simulink model "HVAC"  (R2021a)
settings: Solver=FixedStepAuto  StartTime=0.0  StopTime=1400  FixedStep=1  RelTol=1e-3
values from neighbouring files (symbols this model uses):
  A_w = 1.73    [HVAC_Modeling.m]
  ACCOP = 2.4    [HVAC_Modeling.m]
  AMH = 55    [HVAC_Modeling.m]
  Av = 7.87    [HVAC_Modeling.m]
  c = 1350    [HVAC_Modeling.m]
  Distance = 5.303    [HVAC_Modeling.m]
  h_c = data(2,2:7)    [HVAC_Modeling.m]
  h_v = data(1,2:7)    [HVAC_Modeling.m]
  HCOP = 1    [HVAC_Modeling.m]
  Height = 1.6    [HVAC_Modeling.m]
  m = 0.035    [HVAC_Modeling.m]
  m_a = 0.4    [HVAC_Modeling.m]
  M_a = 3.185    [HVAC_Modeling.m]
  n = 1    [HVAC_Modeling.m]
  R_solar = 0    [HVAC_Modeling.m]
  Tamb = NLT_tem_c(i)    [HVAC_Modeling.m]
  Tc = 23    [HVAC_Modeling.m]
  Ti = NLT_tem_c(i)    [HVAC_Modeling.m]
  Trans = 0.4    [HVAC_Modeling.m]
  Weight = 70    [HVAC_Modeling.m]
settings Model: Creator=LENOVO  LastModifiedBy=LENOVO

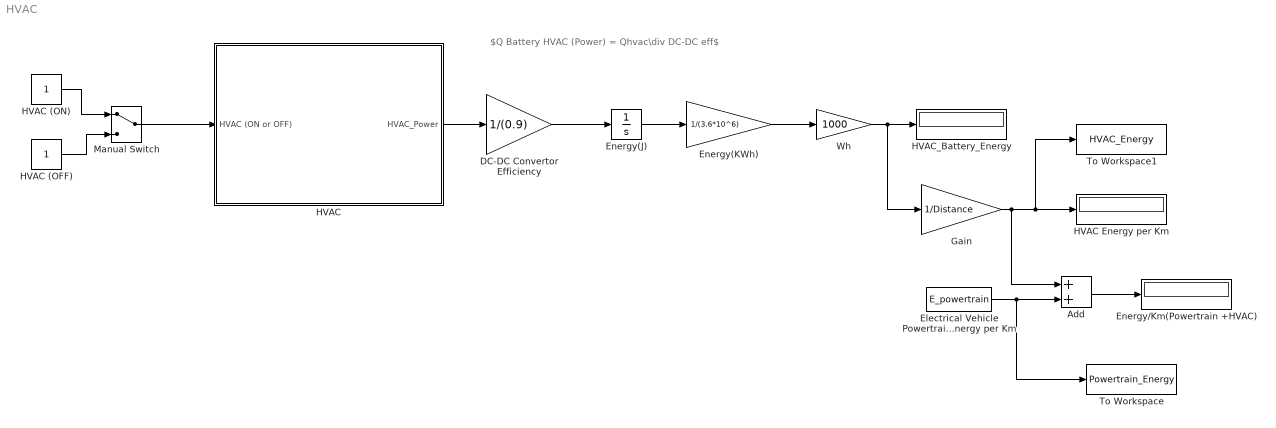
== system HVAC ==
  note: $Q Battery HVAC (Power) = Qhvac\div DC-DC eff$
  Add : Sum
  DC-DC Convertor Efficiency : Gain  Gain=1/(0.9)
  "Electrical Vehicle Powertrain Energy per Km " : FromWorkspace  VariableName=E_powertrain
  Energy(J) : Integrator
  Energy(KWh) : Gain  Gain=1/(3.6*10^6)
  Energy/Km(Powertrain +HVAC) : Display
  Gain : Gain  Gain=1/Distance
  HVAC : Subsystem
  HVAC (OFF) : Constant
  HVAC (ON) : Constant
  HVAC Energy per Km : Display
  HVAC_Battery_Energy : Display
  Manual Switch : ManualSwitch
  To Workspace : ToWorkspace  VariableName=Powertrain_Energy  SaveFormat=Timeseries  SampleTime=-1
  To Workspace1 : ToWorkspace  VariableName=HVAC_Energy  SaveFormat=Timeseries  SampleTime=-1
  Wh : Gain  Gain=1000
  wires:
  HVAC/1(HVAC_Power) -> DC-DC Convertor Efficiency/1
  DC-DC Convertor Efficiency/1 -> Energy(J)/1
  Energy(J)/1 -> Energy(KWh)/1
  Energy(KWh)/1 -> Wh/1
  Wh/1 -> Gain/1, HVAC_Battery_Energy/1
  Gain/1 -> Add/1, To Workspace1/1, HVAC Energy per Km/1
  "Electrical Vehicle Powertrain Energy per Km "/1 -> To Workspace/1, Add/2
  Add/1 -> Energy/Km(Powertrain +HVAC)/1
  Manual Switch/1 -> HVAC/1(HVAC (ON or OFF))
  HVAC (ON)/1 -> Manual Switch/1
  HVAC (OFF)/1 -> Manual Switch/2

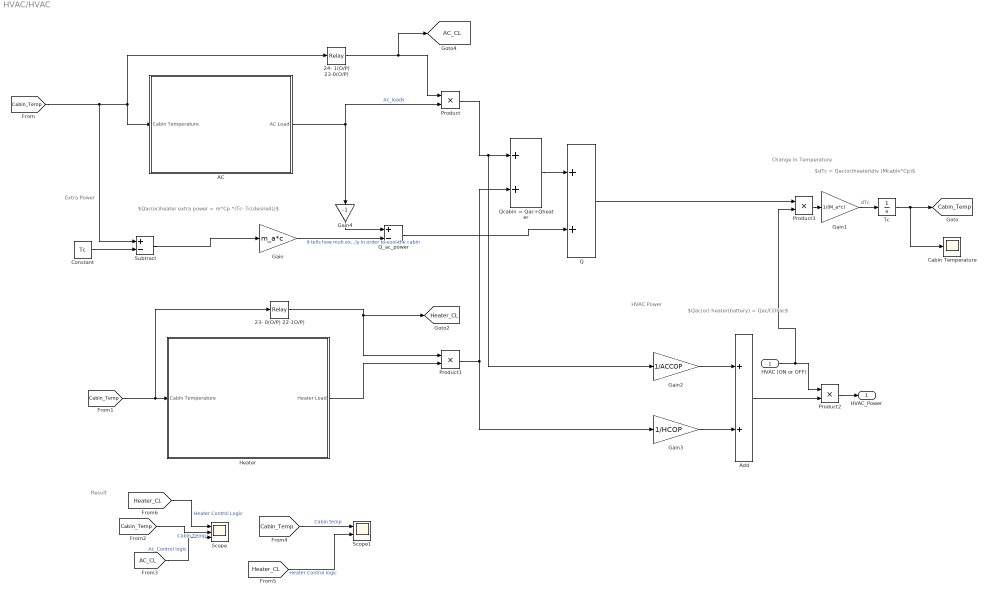
== system HVAC/HVAC ==
  note: HVAC Power
  note: $Qac(or) heater(battery) = Qac/COPac$
  note: Result
  note: Change in Temperature
  note: Extra Power
  note: $dTc = Qac(or)heater\div (Mcabin*Cp)$
  note: $Qac(or)heater extra power = m*Cp *(Tc- Tc(desired))$
  HVAC (ON or OFF) : Inport
  23- 0(O/P) 22-1O/P) : Relay  OnSwitchValue=Tc  OffSwitchValue=Tc-1  OnOutputValue=0  OffOutputValue=1
  24- 1(O/P) 23-0(O/P) : Relay  OnSwitchValue=Tc+1  OffSwitchValue=Tc
  AC : Subsystem
  Add : Sum
  Cabin Temperature : Scope
  Constant : Constant  Value=Tc
  Gain : Gain  Gain=m_a*c
  Gain1 : Gain  Gain=1/(M_a*c)
  Gain2 : Gain  Gain=1/ACCOP
  Gain3 : Gain  Gain=1/HCOP
  Gain4 : Gain  Gain=-1
  Heater : Subsystem
  Product{,1..3} (4 alike) : Product
  Q : Sum
  Q_ac_power : Sum  Inputs=+-
  Qcabin = Qac+Qheater : Sum
  Scope : Scope  NumInputPorts=3
  Scope1 : Scope  NumInputPorts=2
  Subtract : Sum  Inputs=+-
  Tc : Integrator  InitialCondition=Ti
  HVAC_Power : Outport
  tag scope: AC_CL=global, Cabin_Temp=global, Heater_CL=global
  wires:
  Constant/1 -> Subtract/2
  Subtract/1 -> Gain/1
  Gain/1 -> Q_ac_power/2  "It tells how muh extra power need to supply in order to cool the cabin"
  AC/1(AC Load) -> Product/2, Gain4/1  "Ac_loads"
  Gain1/1 -> Tc/1  "dTc"
  [Cabin_Temp] -> AC/1(Cabin Temperature), 24- 1(O/P) 23-0(O/P)/1, Subtract/1
  [Cabin_Temp] -> 23- 0(O/P) 22-1O/P)/1, Heater/1(Cabin Temperature)
  24- 1(O/P) 23-0(O/P)/1 -> [AC_CL], Product/1
  23- 0(O/P) 22-1O/P)/1 -> Product1/1, [Heater_CL]
  Heater/1(Heater Load) -> Product1/2
  Product/1 -> Qcabin = Qac+Qheater/1, Gain2/1
  Qcabin = Qac+Qheater/1 -> Q/1
  Q_ac_power/1 -> Q/2
  Tc/1 -> Cabin Temperature/1, [Cabin_Temp]
  [Cabin_Temp] -> Scope/2  "Cabin Temp"
  [AC_CL] -> Scope/3  "Ac_Control logic"
  [Cabin_Temp] -> Scope1/1  "Cabin temp"
  [Heater_CL] -> Scope1/2  "Heater Control logic"
  Product1/1 -> Gain3/1, Qcabin = Qac+Qheater/2
  Gain2/1 -> Add/1
  Gain3/1 -> Add/2
  Gain4/1 -> Q_ac_power/1
  Add/1 -> Product2/2
  HVAC (ON or OFF)/1 -> Product3/2, Product2/1
  Product2/1 -> HVAC_Power/1
  Product3/1 -> Gain1/1
  Q/1 -> Product3/1
  [Heater_CL] -> Scope/1  "Heater Control Logic"

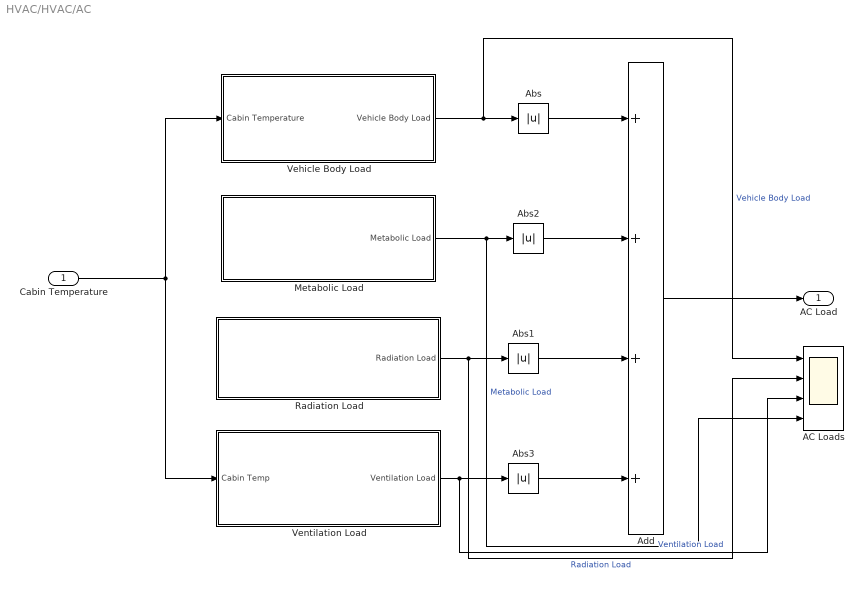
== system HVAC/HVAC/AC ==
  Cabin Temperature : Inport
  AC Loads : Scope  NumInputPorts=4
  Abs{,1..3} (4 alike) : Abs
  Add : Sum  Inputs=++++
  Metabolic Load : Subsystem
  Radiation Load : Subsystem
  Vehicle Body Load : Subsystem
  Ventilation Load : Subsystem
  AC Load : Outport
  wires:
  Cabin Temperature/1 -> Vehicle Body Load/1(Cabin Temperature), Ventilation Load/1(Cabin Temp)
  Metabolic Load/1(Metabolic Load) -> AC Loads/4, Abs2/1  "Metabolic Load"
  Add/1 -> AC Load/1
  Vehicle Body Load/1(Vehicle Body Load) -> AC Loads/1, Abs/1  "Vehicle Body Load"
  Abs/1 -> Add/1
  Abs2/1 -> Add/2
  Radiation Load/1(Radiation Load) -> AC Loads/2, Abs1/1  "Radiation Load"
  Abs1/1 -> Add/3
  Ventilation Load/1(Ventilation Load) -> AC Loads/3, Abs3/1  "Ventilation Load"
  Abs3/1 -> Add/4

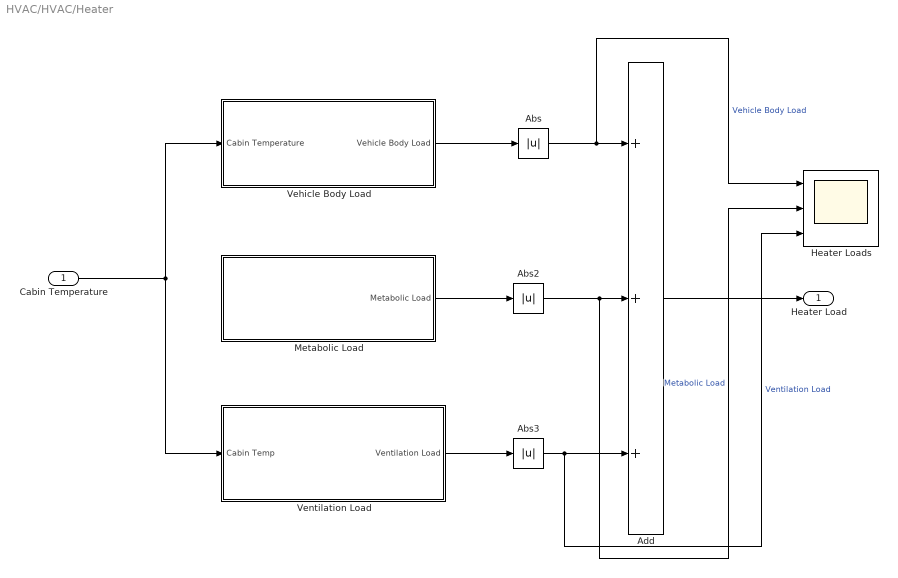
== system HVAC/HVAC/Heater ==
  Cabin Temperature : Inport
  Abs : Abs
  Abs2 : Abs
  Abs3 : Abs
  Add : Sum  Inputs=+++
  Heater Loads : Scope  NumInputPorts=3
  Metabolic Load : Subsystem
  Vehicle Body Load : Subsystem
  Ventilation Load : Subsystem
  Heater Load : Outport
  wires:
  Cabin Temperature/1 -> Vehicle Body Load/1(Cabin Temperature), Ventilation Load/1(Cabin Temp)
  Metabolic Load/1(Metabolic Load) -> Abs2/1
  Add/1 -> Heater Load/1
  Vehicle Body Load/1(Vehicle Body Load) -> Abs/1
  Abs/1 -> Heater Loads/1, Add/1  "Vehicle Body Load"
  Abs2/1 -> Heater Loads/2, Add/2  "Metabolic Load"
  Ventilation Load/1(Ventilation Load) -> Abs3/1
  Abs3/1 -> Heater Loads/3, Add/3  "Ventilation Load"

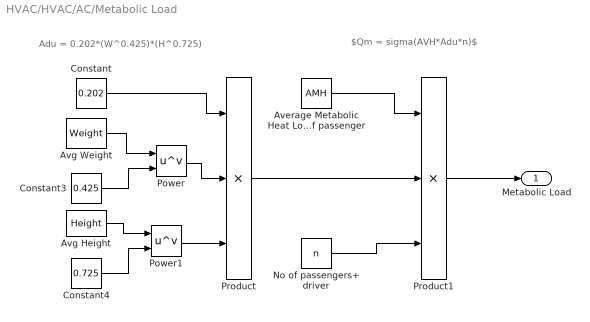
== system HVAC/HVAC/AC/Metabolic Load ==
  note: Adu = 0.202*(W^0.425)*(H^0.725)
  note: $Qm = sigma(AVH*Adu*n)$
  Average Metabolic Heat Load of passenger : Constant  Value=AMH
  Avg Height : Constant  Value=Height
  Avg Weight : Constant  Value=Weight
  Constant : Constant  Value=0.202
  Constant3 : Constant  Value=0.425
  Constant4 : Constant  Value=0.725
  "No of passengers+ driver " : Constant  Value=n
  Power : Math  Operator=pow  SaturateOnIntegerOverflow=on
  Power1 : Math  Operator=pow  SaturateOnIntegerOverflow=on
  Product : Product  Inputs=3
  Product1 : Product  Inputs=3
  Metabolic Load : Outport
  wires:
  Constant/1 -> Product/1
  Avg Weight/1 -> Power/1
  Constant3/1 -> Power/2
  Avg Height/1 -> Power1/1
  Constant4/1 -> Power1/2
  Power1/1 -> Product/3
  Power/1 -> Product/2
  Product/1 -> Product1/2
  Average Metabolic Heat Load of passenger/1 -> Product1/1
  "No of passengers+ driver "/1 -> Product1/3
  Product1/1 -> Metabolic Load/1

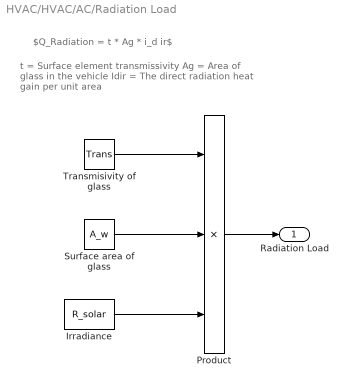
== system HVAC/HVAC/AC/Radiation Load ==
  note: t = Surface element transmissivity
      | Ag = Area of glass in the vehicle
      | Idir = The direct radiation heat gain per unit area
  note: $Q_Radiation = t * Ag * i_d ir$
  Irradiance : Constant  Value=R_solar
  Product : Product  Inputs=3
  Surface area of glass : Constant  Value=A_w
  Transmisivity of glass : Constant  Value=Trans
  Radiation Load : Outport
  wires:
  Transmisivity of glass/1 -> Product/1
  Irradiance/1 -> Product/3
  Surface area of glass/1 -> Product/2
  Product/1 -> Radiation Load/1

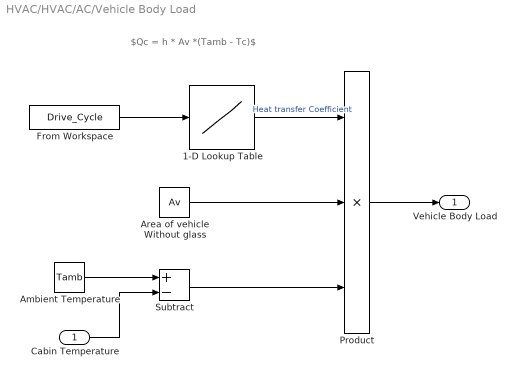
== system HVAC/HVAC/AC/Vehicle Body Load ==
  note: $Qc = h * Av *(Tamb - Tc)$
  Cabin Temperature : Inport
  1-D Lookup Table : Lookup_n-D  NumberOfTableDimensions=1  BreakpointsForDimension1=h_v  Table=h_c  InternalRulePriority=Speed  RndMeth=Simplest  InputSameDT=on
  Ambient Temperature : Constant  Value=Tamb
  Area of vehicle Without glass : Constant  Value=Av
  From Workspace : FromWorkspace  VariableName=Drive_Cycle
  Product : Product  Inputs=3
  Subtract : Sum  Inputs=+-
  Vehicle Body Load : Outport
  wires:
  From Workspace/1 -> 1-D Lookup Table/1
  Ambient Temperature/1 -> Subtract/1
  Cabin Temperature/1 -> Subtract/2
  1-D Lookup Table/1 -> Product/1  "Heat transfer Coefficient"
  Area of vehicle Without glass/1 -> Product/2
  Subtract/1 -> Product/3
  Product/1 -> Vehicle Body Load/1

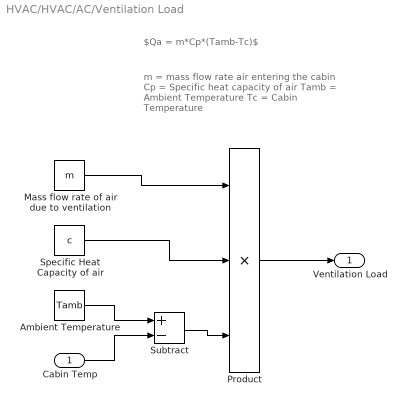
== system HVAC/HVAC/AC/Ventilation Load ==
  note: m = mass flow rate air entering the cabin
      | Cp = Specific heat capacity of air
      | Tamb = Ambient Temperature
      | Tc = Cabin Temperature
  note: $Qa = m*Cp*(Tamb-Tc)$
  Cabin Temp : Inport
  Ambient Temperature : Constant  Value=Tamb
  "Mass flow rate of air due to ventilation " : Constant  Value=m
  Product : Product  Inputs=3
  Specific Heat Capacity of air : Constant  Value=c
  Subtract : Sum  Inputs=+-
  Ventilation Load : Outport
  wires:
  Ambient Temperature/1 -> Subtract/1
  Cabin Temp/1 -> Subtract/2
  "Mass flow rate of air due to ventilation "/1 -> Product/1
  Specific Heat Capacity of air/1 -> Product/2
  Subtract/1 -> Product/3
  Product/1 -> Ventilation Load/1

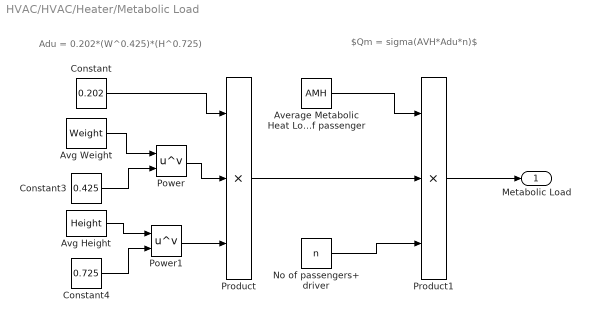
== system HVAC/HVAC/Heater/Metabolic Load ==
  note: Adu = 0.202*(W^0.425)*(H^0.725)
  note: $Qm = sigma(AVH*Adu*n)$
  Average Metabolic Heat Load of passenger : Constant  Value=AMH
  Avg Height : Constant  Value=Height
  Avg Weight : Constant  Value=Weight
  Constant : Constant  Value=0.202
  Constant3 : Constant  Value=0.425
  Constant4 : Constant  Value=0.725
  "No of passengers+ driver " : Constant  Value=n
  Power : Math  Operator=pow  SaturateOnIntegerOverflow=on
  Power1 : Math  Operator=pow  SaturateOnIntegerOverflow=on
  Product : Product  Inputs=3
  Product1 : Product  Inputs=3
  Metabolic Load : Outport
  wires:
  Constant/1 -> Product/1
  Avg Weight/1 -> Power/1
  Constant3/1 -> Power/2
  Avg Height/1 -> Power1/1
  Constant4/1 -> Power1/2
  Power1/1 -> Product/3
  Power/1 -> Product/2
  Product/1 -> Product1/2
  Average Metabolic Heat Load of passenger/1 -> Product1/1
  "No of passengers+ driver "/1 -> Product1/3
  Product1/1 -> Metabolic Load/1

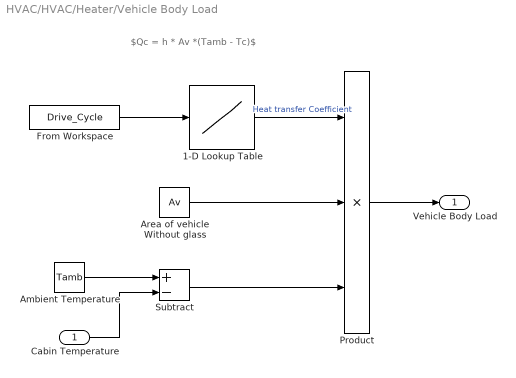
== system HVAC/HVAC/Heater/Vehicle Body Load ==
  note: $Qc = h * Av *(Tamb - Tc)$
  Cabin Temperature : Inport
  1-D Lookup Table : Lookup_n-D  NumberOfTableDimensions=1  BreakpointsForDimension1=h_v  Table=h_c  InternalRulePriority=Speed  RndMeth=Simplest  InputSameDT=on
  Ambient Temperature : Constant  Value=Tamb
  Area of vehicle Without glass : Constant  Value=Av
  From Workspace : FromWorkspace  VariableName=Drive_Cycle
  Product : Product  Inputs=3
  Subtract : Sum  Inputs=+-
  Vehicle Body Load : Outport
  wires:
  From Workspace/1 -> 1-D Lookup Table/1
  Ambient Temperature/1 -> Subtract/1
  Cabin Temperature/1 -> Subtract/2
  1-D Lookup Table/1 -> Product/1  "Heat transfer Coefficient"
  Area of vehicle Without glass/1 -> Product/2
  Subtract/1 -> Product/3
  Product/1 -> Vehicle Body Load/1

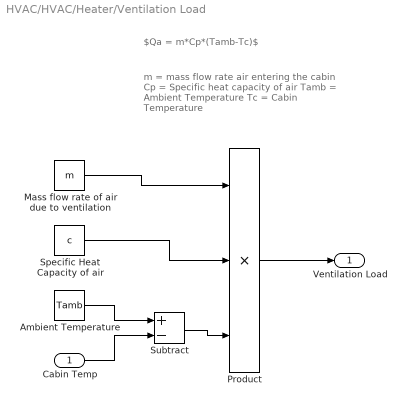
== system HVAC/HVAC/Heater/Ventilation Load ==
  note: m = mass flow rate air entering the cabin
      | Cp = Specific heat capacity of air
      | Tamb = Ambient Temperature
      | Tc = Cabin Temperature
  note: $Qa = m*Cp*(Tamb-Tc)$
  Cabin Temp : Inport
  Ambient Temperature : Constant  Value=Tamb
  "Mass flow rate of air due to ventilation " : Constant  Value=m
  Product : Product  Inputs=3
  Specific Heat Capacity of air : Constant  Value=c
  Subtract : Sum  Inputs=+-
  Ventilation Load : Outport
  wires:
  Ambient Temperature/1 -> Subtract/1
  Cabin Temp/1 -> Subtract/2
  "Mass flow rate of air due to ventilation "/1 -> Product/1
  Specific Heat Capacity of air/1 -> Product/2
  Subtract/1 -> Product/3
  Product/1 -> Ventilation Load/1
